simulink library "ADC_labels_lib"  (Simulink 7.2)
settings: Solver=ode45  SolverMode=SingleTasking  StartTime=0.0  StopTime=10.0  RelTol=1e-3
libraries: simulink x1
settings Model: Creator=cbuttril  LastModifiedBy=amurch

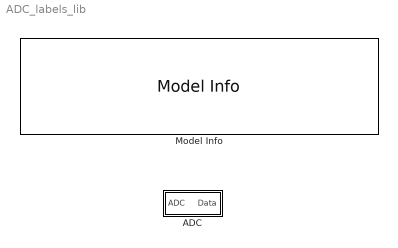
== system ADC_labels_lib ==
  ADC : Subsystem
  Model Info : simulink/Model-Wide Utilities/Model Info  SystemSampleTime=-1  InitialBlockCM=None  BlockCM=None  Frame=on  DisplayStringWithTags=|  HorizontalTextAlignment=Center  LeftAlignmentValue=0.5  SourceBlockDiagram=ADC_labels_lib  TagMaxNumber=20
      | Developed using Matlab Release 2007a
      | 
      | SVN:%<ModelVersion>
      | Last modifed by %<LastModifiedBy> on %<LastModificationDate>

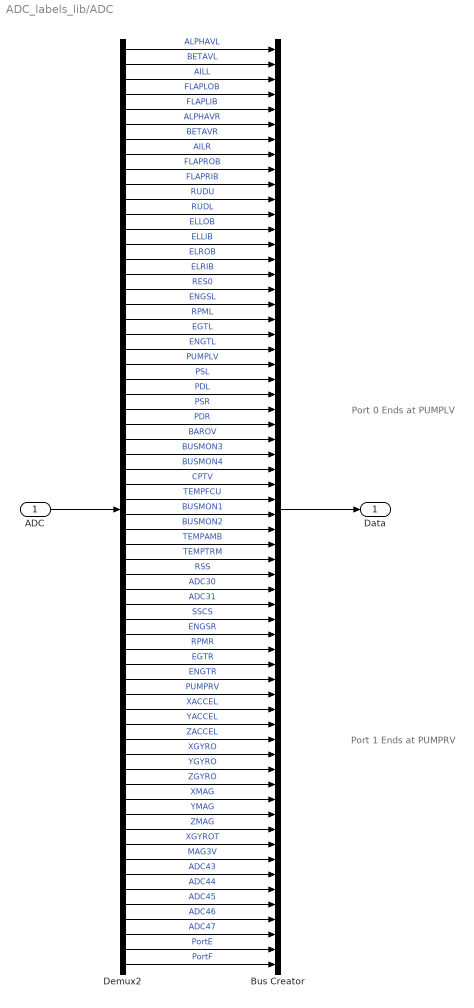
== system ADC_labels_lib/ADC ==
  note: Port 1 Ends at PUMPRV
  note: Port 0 Ends at PUMPLV
  ADC : Inport  PortDimensions=62  OutDataType=sfix(16)  OutScaling=2^0
  Bus Creator : BusCreator  Inputs=62
  Demux2 : Demux  Outputs=62
  Data : Outport  PortDimensions=62  OutDataType=sfix(16)  OutScaling=2^0
  wires:
  Bus Creator/1 -> Data/1
  ADC/1 -> Demux2/1
  Demux2/1 -> Bus Creator/1  "ALPHAVL"
  Demux2/2 -> Bus Creator/2  "BETAVL"
  Demux2/3 -> Bus Creator/3  "AILL"
  Demux2/4 -> Bus Creator/4  "FLAPLOB"
  Demux2/5 -> Bus Creator/5  "FLAPLIB"
  Demux2/6 -> Bus Creator/6  "ALPHAVR"
  Demux2/7 -> Bus Creator/7  "BETAVR"
  Demux2/8 -> Bus Creator/8  "AILR"
  Demux2/9 -> Bus Creator/9  "FLAPROB"
  Demux2/10 -> Bus Creator/10  "FLAPRIB"
  Demux2/11 -> Bus Creator/11  "RUDU"
  Demux2/12 -> Bus Creator/12  "RUDL"
  Demux2/13 -> Bus Creator/13  "ELLOB"
  Demux2/14 -> Bus Creator/14  "ELLIB"
  Demux2/15 -> Bus Creator/15  "ELROB"
  Demux2/16 -> Bus Creator/16  "ELRIB"
  Demux2/17 -> Bus Creator/17  "RES0"
  Demux2/18 -> Bus Creator/18  "ENGSL"
  Demux2/19 -> Bus Creator/19  "RPML"
  Demux2/20 -> Bus Creator/20  "EGTL"
  Demux2/21 -> Bus Creator/21  "ENGTL"
  Demux2/22 -> Bus Creator/22  "PUMPLV"
  Demux2/23 -> Bus Creator/23  "PSL"
  Demux2/24 -> Bus Creator/24  "PDL"
  Demux2/25 -> Bus Creator/25  "PSR"
  Demux2/26 -> Bus Creator/26  "PDR"
  Demux2/27 -> Bus Creator/27  "BAROV"
  Demux2/28 -> Bus Creator/28  "BUSMON3"
  Demux2/29 -> Bus Creator/29  "BUSMON4"
  Demux2/30 -> Bus Creator/30  "CPTV"
  Demux2/31 -> Bus Creator/31  "TEMPFCU"
  Demux2/32 -> Bus Creator/32  "BUSMON1"
  Demux2/33 -> Bus Creator/33  "BUSMON2"
  Demux2/34 -> Bus Creator/34  "TEMPAMB"
  Demux2/35 -> Bus Creator/35  "TEMPTRM"
  Demux2/36 -> Bus Creator/36  "RSS"
  Demux2/37 -> Bus Creator/37  "ADC30"
  Demux2/38 -> Bus Creator/38  "ADC31"
  Demux2/39 -> Bus Creator/39  "SSCS"
  Demux2/40 -> Bus Creator/40  "ENGSR"
  Demux2/41 -> Bus Creator/41  "RPMR"
  Demux2/42 -> Bus Creator/42  "EGTR"
  Demux2/43 -> Bus Creator/43  "ENGTR"
  Demux2/44 -> Bus Creator/44  "PUMPRV"
  Demux2/45 -> Bus Creator/45  "XACCEL"
  Demux2/46 -> Bus Creator/46  "YACCEL"
  Demux2/47 -> Bus Creator/47  "ZACCEL"
  Demux2/48 -> Bus Creator/48  "XGYRO"
  Demux2/49 -> Bus Creator/49  "YGYRO"
  Demux2/50 -> Bus Creator/50  "ZGYRO"
  Demux2/51 -> Bus Creator/51  "XMAG"
  Demux2/52 -> Bus Creator/52  "YMAG"
  Demux2/53 -> Bus Creator/53  "ZMAG"
  Demux2/54 -> Bus Creator/54  "XGYROT"
  Demux2/55 -> Bus Creator/55  "MAG3V"
  Demux2/56 -> Bus Creator/56  "ADC43"
  Demux2/57 -> Bus Creator/57  "ADC44"
  Demux2/58 -> Bus Creator/58  "ADC45"
  Demux2/59 -> Bus Creator/59  "ADC46"
  Demux2/60 -> Bus Creator/60  "ADC47"
  Demux2/61 -> Bus Creator/61  "PortE"
  Demux2/62 -> Bus Creator/62  "PortF"
